simulink model "raw2jointtest"  (R2016a)
settings: Solver=ode5  StartTime=0.0  StopTime=inf  FixedStep=0.001  RelTol=1e-3
libraries: dcpctrl x3
settings Model: SimulationMode=external  Creator=julianleland  LastModifiedBy=julianleland
settings HardwareCC: ProdBitPerLong=64  ProdLargestAtomicFloat=None  ProdHWDeviceType=Intel->x86-64  TargetBitPerLong=64  TargetBitPerPointer=64  TargetIntDivRoundTo=Zero  TargetEndianess=LittleEndian  TargetWordSize=64  TargetHWDeviceType=Intel->x86-64
settings RTWCC: SystemTargetFile=sldrt.tlc  TemplateMakefile=sldrt.tmf  Description=Simulink Desktop Real-Time  RTWCompilerOptimization=on
settings CodeAppCC: MaxIdLength=95
settings SimulinkDesktopRealTimeCC: TargetPreCompLibLocation=/Applications/MATLAB_R2016a.app/toolbox/sldrt/lib/maci64  TargetLangStandard=C89/C90 (ANSI)  SupportVariableSizeSignals=off

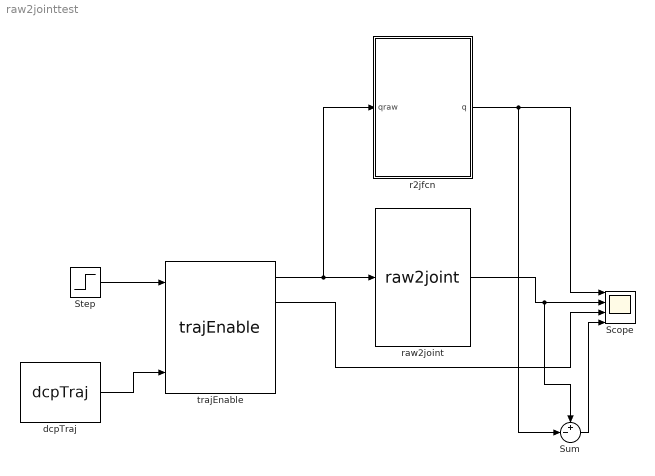
== system raw2jointtest ==
  Scope : Scope  NumInputPorts=4
  Step : Step  SampleTime=0
  Sum : Sum  Inputs=+-|
  dcpTraj : dcpctrl/dcpTraj
  r2jfcn : Subsystem
  raw2joint : dcpctrl/raw2joint
  trajEnable : dcpctrl/trajEnable
  wires:
  trajEnable/2 -> Scope/3
  raw2joint/1 -> Sum/1, Scope/2
  Sum/1 -> Scope/4
  dcpTraj/1 -> trajEnable/3
  Step/1 -> trajEnable/1
  trajEnable/1 -> r2jfcn/1(qraw), raw2joint/1
  r2jfcn/1(q) -> Sum/2, Scope/1

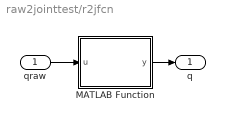
== system raw2jointtest/r2jfcn ==
  qraw : Inport
  MATLAB Function : MATLAB Function  TreatAsAtomicUnit=on
  q : Outport
  wires:
  MATLAB Function/1(y) -> q/1
  qraw/1 -> MATLAB Function/1(u)

== matlab function raw2jointtest/r2jfcn/MATLAB Function ==
  data: u input; y output; robot parameter
function y = fcn(u, robot)
%#codegen

y_temp = r2jfcn(u(1),u(2),u(3),u(4));
y = y_temp';
